simulink model "dbe_xaui_corr_32X"  (Simulink 7.1)
settings: Solver=ode45  StartTime=0.0  StopTime=1000  RelTol=1e-3
undefined symbols (not defined in the file or in its folder): iBOB
libraries: xbsIndex_r4 x455, xps_library x46, casper_library_misc x12, casper_library_sources x2, gavrt_library x1, simulink x1, casper_library_scopes x1
(part 2 of 4)

== system dbe_xaui_corr_32X/onepps_sync ==
  ext_1pps : Inport  OutDataType=sfix(16)  OutScaling=2^0
  Step : Step  Time=200  Before=1  After=0  SampleTime=1
  Terminator : Terminator
  arm1pps : xps_library/software register  Tag=xps:sw_reg  SystemSampleTime=-1  io_dir=From Processor  arith_type=Unsigned  bitwidth=32  bin_pt=0  sample_period=1  gw_name=dbe_xaui_corr_32X_onepps_sync_arm1pps_user_data_out
      link override dbe_xaui_corr_32X_onepps_sync_arm1pps_user_data_out: arith_type=Unsigned  n_bits=32  bin_pt=0  period=1
      link override dbe_xaui_corr_onepps_sync_arm1pps_user_data_out: arith_type=Unsigned  n_bits=32  bin_pt=0  period=1
      link override dbe_xaui_onepps_sync_arm1pps_user_data_out: arith_type=Unsigned  n_bits=32  bin_pt=0  period=1
      link override vlbipfb2_m3_ibob_onepps_sync_arm1pps_user_data_out: arith_type=Unsigned  n_bits=32  bin_pt=0  period=1
      link override vlbipfb2_m3_roach_onepps_sync_arm1pps_user_data_out: arith_type=Unsigned  n_bits=32  bin_pt=0  period=1
  arm1pps_ack : xps_library/software register  Tag=xps:sw_reg  SystemSampleTime=-1  io_dir=To Processor  arith_type=Unsigned  bitwidth=32  bin_pt=0  sample_period=1  gw_name=dbe_xaui_corr_32X_onepps_sync_arm1pps_ack_user_data_in
      link override convert: arith_type=Unsigned  n_bits=32  bin_pt=0
  armshake : Subsystem
  int_1pps_gen : Subsystem
  int_1pps : Outport  OutDataType=sfix(16)  OutScaling=2^0
  wires:
  int_1pps_gen/1(1pps) -> int_1pps/1
  ext_1pps/1 -> armshake/1(ext_1pps)
  arm1pps/1 -> armshake/2(ext_arm1pps)
  Step/1 -> arm1pps/1
  armshake/1(rst_1pps) -> int_1pps_gen/1(rst)
  armshake/2(arm_ack) -> arm1pps_ack/1
  arm1pps_ack/1 -> Terminator/1

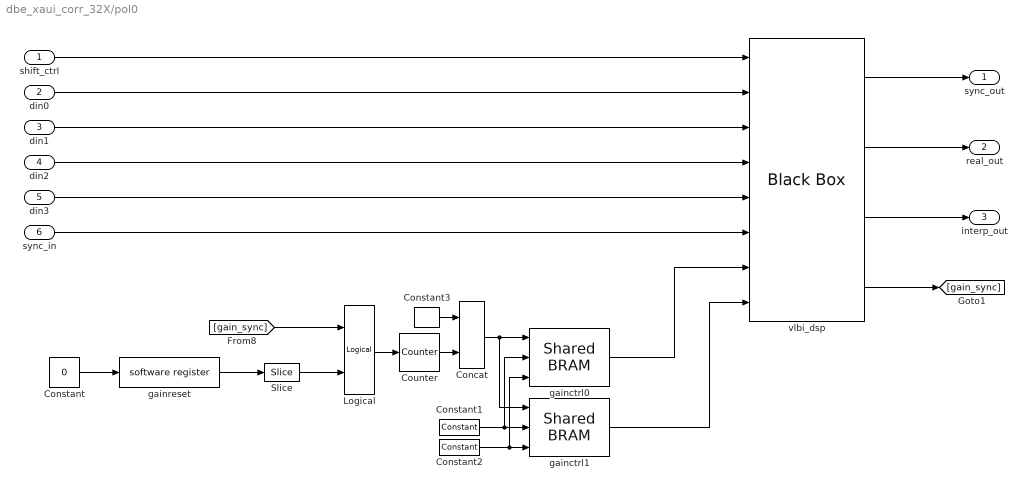
== system dbe_xaui_corr_32X/pol0 ==
  shift_ctrl : Inport  OutDataType=sfix(16)  OutScaling=2^0
  din0 : Inport  Port=2  OutDataType=sfix(16)  OutScaling=2^0
  din1 : Inport  Port=3  OutDataType=sfix(16)  OutScaling=2^0
  din2 : Inport  Port=4  OutDataType=sfix(16)  OutScaling=2^0
  din3 : Inport  Port=5  OutDataType=sfix(16)  OutScaling=2^0
  sync_in : Inport  Port=6  OutDataType=sfix(16)  OutScaling=2^0
  Concat : xbsIndex_r4/Concat  num_inputs=2  dbl_ovrd=off  block_type=concat
      settings: block_version=11.3
  Constant : Constant  Value=0  OutDataType=sfix(16)  OutScaling=2^0
  Constant1 : xbsIndex_r4/Constant  arith_type=Unsigned  const=0  n_bits=32  bin_pt=0  explicit_period=on  period=1  equ=P=C  opselect=C  inp2=PCIN>>17  opr=+  inp1=P  carry=CIN  dbl_ovrd=off  block_type=constant
      settings: block_version=11.3
  Constant2 : xbsIndex_r4/Constant  arith_type=Boolean  const=0  n_bits=1  bin_pt=0  explicit_period=on  period=1  equ=P=C  opselect=C  inp2=PCIN>>17  opr=+  inp1=P  carry=CIN  dbl_ovrd=off  block_type=constant
      settings: block_version=11.3
  Constant3 : xbsIndex_r4/Constant  arith_type=Unsigned  const=0  n_bits=8  bin_pt=0  explicit_period=on  period=1  equ=P=C  opselect=C  inp2=PCIN>>17  opr=+  inp1=P  carry=CIN  dbl_ovrd=off  block_type=constant
      settings: block_version=11.3
  Counter : xbsIndex_r4/Counter  cnt_type=Free Running  cnt_to=Inf  operation=Up  start_count=0  cnt_by_val=1  arith_type=Unsigned  n_bits=3  bin_pt=0  load_pin=off  rst=on  en=off  explicit_period=off  period=1  dbl_ovrd=off  use_behavioral_HDL=off  use_rpm=on  implementation=Fabric  block_type=counter
      settings: xl_area=[0, 0, 0, 0, 0, 0, 0]  block_version=11.3
  Logical : xbsIndex_r4/Logical  logical_function=OR  inputs=2  en=off  latency=0  precision=Full  arith_type=Unsigned  n_bits=8  bin_pt=2  align_bp=on  dbl_ovrd=off  block_type=logical
      settings: xl_area=[0, 0, 0, 0, 0, 0, 0]  block_version=11.3
  Slice : xbsIndex_r4/Slice  nbits=1  boolean_output=on  mode=Lower Bit Location + Width  bit1=0  base1=MSB of Input  bit0=0  base0=LSB of Input  dbl_ovrd=off  block_type=slice
      settings: block_version=11.3
  gainctrl0 : xps_library/Shared BRAM  Tag=xps:bram  SystemSampleTime=-1  arith_type="Signed  (2's comp)"  addr_width=11  data_width=32  data_bin_pt=0  init_vals=[0 0 100 0 zeros(1,2^11-4)]  sample_rate=1
      link override convert_din: arith_type="Signed  (2's comp)"
      link override dbe_adc_single_pol0_gainctrl0_data_out: arith_type="Signed  (2's comp)"
      link override dbe_xaui_corr_32X_pol0_gainctrl0_data_out: arith_type="Signed  (2's comp)"
      link override mem/sim_data_in: arith_type="Signed  (2's comp)"
      link override vlbipfb2_m3_ibob_pol0_gainctrl0_data_out: arith_type="Signed  (2's comp)"
      link override vlbipfb2_m3_roach_pol0_gainctrl0_data_out: arith_type="Signed  (2's comp)"
  gainctrl1 : xps_library/Shared BRAM  Tag=xps:bram  SystemSampleTime=-1  arith_type="Signed  (2's comp)"  addr_width=11  data_width=32  data_bin_pt=0  init_vals=zeros(1,2^11)  sample_rate=1
      link override convert_din: arith_type="Signed  (2's comp)"
      link override dbe_adc_single_pol0_gainctrl1_data_out: arith_type="Signed  (2's comp)"
      link override dbe_xaui_corr_32X_pol0_gainctrl1_data_out: arith_type="Signed  (2's comp)"
      link override mem/sim_data_in: arith_type="Signed  (2's comp)"
      link override vlbipfb2_m3_ibob_pol0_gainctrl1_data_out: arith_type="Signed  (2's comp)"
      link override vlbipfb2_m3_roach_pol0_gainctrl1_data_out: arith_type="Signed  (2's comp)"
  gainreset : xps_library/software register  Tag=xps:sw_reg  SystemSampleTime=-1  io_dir=From Processor  arith_type=Unsigned  bitwidth=32  bin_pt=0  sample_period=1  gw_name=dbe_xaui_corr_32X_pol0_gainreset_user_data_out
      link override dbe_adc_single_pol0_gainreset_user_data_out: arith_type=Unsigned  n_bits=32  bin_pt=0  period=1
      link override dbe_xaui_corr_32X_pol0_gainreset_user_data_out: arith_type=Unsigned  n_bits=32  bin_pt=0  period=1
      link override vlbipfb2_m3_ibob_pol0_gainreset_user_data_out: arith_type=Unsigned  n_bits=32  bin_pt=0  period=1
      link override vlbipfb2_m3_roach_pol0_gainreset_user_data_out: arith_type=Unsigned  n_bits=32  bin_pt=0  period=1
  vlbi_dsp : xbsIndex_r4/Black Box  init_code=vlbi_dsp_core_config  sim_method=Inactive  block_type=blackbox2
      settings: infoedit="Incorporates black box HDL and simulation model into a System Generator design.<P><P>You must supply a Black Box with certain information about the HDL component you would like to bring into System Generator. This information is provided through a Matlab function.<P><P>When \"Simulation mode\" is set to \"Inactive\", you will typically want to provide a separate simulation model by using a Simulation Multiplexer.<P>When \"Simulation mode\" is set to \"External co-simulator\", you must include a ModelSim block in the design."  block_version=10.1.3
  sync_out : Outport  OutDataType=sfix(16)  OutScaling=2^0
  real_out : Outport  Port=2  OutDataType=sfix(16)  OutScaling=2^0
  interp_out : Outport  Port=3  OutDataType=sfix(16)  OutScaling=2^0
  wires:
  Constant3/1 -> Concat/1
  Counter/1 -> Concat/2
  Concat/1 -> gainctrl0/1, gainctrl1/1
  Constant1/1 -> gainctrl0/2, gainctrl1/2
  Constant2/1 -> gainctrl1/3, gainctrl0/3
  Constant/1 -> gainreset/1
  Logical/1 -> Counter/1
  gainreset/1 -> Slice/1
  Slice/1 -> Logical/2
  shift_ctrl/1 -> vlbi_dsp/1
  din0/1 -> vlbi_dsp/2
  din1/1 -> vlbi_dsp/3
  din2/1 -> vlbi_dsp/4
  din3/1 -> vlbi_dsp/5
  sync_in/1 -> vlbi_dsp/6
  gainctrl0/1 -> vlbi_dsp/7
  gainctrl1/1 -> vlbi_dsp/8
  vlbi_dsp/1 -> sync_out/1
  vlbi_dsp/2 -> real_out/1
  vlbi_dsp/3 -> interp_out/1
  [gain_sync] -> Logical/1
  vlbi_dsp/4 -> [gain_sync]

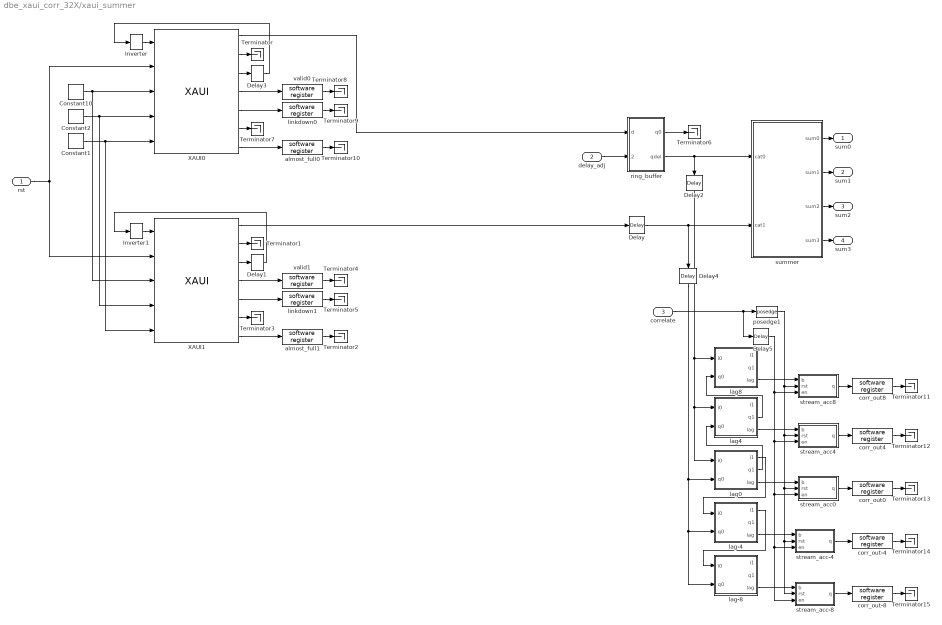
== system dbe_xaui_corr_32X/xaui_summer ==
  rst : Inport  OutDataType=sfix(16)  OutScaling=2^0
  delay_adj : Inport  Port=2  OutDataType=sfix(16)  OutScaling=2^0
  correlate : Inport  Port=3  OutDataType=sfix(16)  OutScaling=2^0
  Constant1 : xbsIndex_r4/Constant  arith_type=Boolean  const=0  n_bits=4  bin_pt=0  explicit_period=on  period=1  equ=P=C  opselect=C  inp2=PCIN>>17  opr=+  inp1=P  carry=CIN  dbl_ovrd=off  block_type=constant
      settings: block_version=11.3
  Constant10 : xbsIndex_r4/Constant  arith_type=Unsigned  const=2^4 -1  n_bits=32  bin_pt=0  explicit_period=on  period=1  equ=P=C  opselect=C  inp2=PCIN>>17  opr=+  inp1=P  carry=CIN  dbl_ovrd=off  block_type=constant
      settings: block_version=11.3
  Constant2 : xbsIndex_r4/Constant  arith_type=Unsigned  const=0  n_bits=4  bin_pt=0  explicit_period=on  period=1  equ=P=C  opselect=C  inp2=PCIN>>17  opr=+  inp1=P  carry=CIN  dbl_ovrd=off  block_type=constant
      settings: block_version=11.3
  Delay : xbsIndex_r4/Delay  en=off  latency=8  dbl_ovrd=off  reg_retiming=on  block_type=delay
  Delay1 : xbsIndex_r4/Delay  en=off  latency=32  dbl_ovrd=off  reg_retiming=off  block_type=delay
      settings: block_version=11.3
  Delay2 : xbsIndex_r4/Delay  Orientation=down  en=off  latency=8  dbl_ovrd=off  reg_retiming=on  block_type=delay
  Delay3 : xbsIndex_r4/Delay  en=off  latency=32  dbl_ovrd=off  reg_retiming=off  block_type=delay
      settings: block_version=11.3
  Delay4 : xbsIndex_r4/Delay  Orientation=down  en=off  latency=8  dbl_ovrd=off  reg_retiming=on  block_type=delay
  Delay5 : xbsIndex_r4/Delay  en=off  latency=2  dbl_ovrd=off  reg_retiming=on  block_type=delay
  Inverter : xbsIndex_r4/Inverter  en=off  latency=0  dbl_ovrd=off  block_type=inv
      settings: block_version=11.3
  Inverter1 : xbsIndex_r4/Inverter  en=off  latency=0  dbl_ovrd=off  block_type=inv
      settings: block_version=11.3
  Terminator{,1..15} (16 alike) : Terminator
  XAUI0 : xps_library/XAUI  Tag=xps:xaui  SystemSampleTime=-1  demux=2  port=iBOB:0  open_phy=off  show_param=off  pre_emph=3  swing=800
      link override convert_tx_data: n_bits=32
      link override convert_tx_outofband: n_bits=4
      link override dbe_xaui_corr_32X_xaui_summer_XAUI0_rx_data: n_bits=32
      link override dbe_xaui_corr_32X_xaui_summer_XAUI0_rx_outofband: n_bits=4
      link override dbe_xaui_corr_xaui_summer_XAUI0_rx_data: n_bits=32
      link override dbe_xaui_corr_xaui_summer_XAUI0_rx_outofband: n_bits=4
      link override dbe_xaui_xaui_summer_XAUI0_rx_data: n_bits=32
      link override dbe_xaui_xaui_summer_XAUI0_rx_outofband: n_bits=4
      link override xaui_XAUI_RECV_rx_data: n_bits=32
      link override xaui_XAUI_RECV_rx_outofband: n_bits=4
  XAUI1 : xps_library/XAUI  Tag=xps:xaui  SystemSampleTime=-1  demux=2  port=iBOB:1  open_phy=off  show_param=off  pre_emph=3  swing=800
      link override convert_tx_data: n_bits=32
      link override convert_tx_outofband: n_bits=4
      link override dbe_xaui_corr_32X_xaui_summer_XAUI1_rx_data: n_bits=32
      link override dbe_xaui_corr_32X_xaui_summer_XAUI1_rx_outofband: n_bits=4
      link override dbe_xaui_corr_xaui_summer_XAUI1_rx_data: n_bits=32
      link override dbe_xaui_corr_xaui_summer_XAUI1_rx_outofband: n_bits=4
      link override dbe_xaui_xaui_summer_XAUI1_rx_data: n_bits=32
      link override dbe_xaui_xaui_summer_XAUI1_rx_outofband: n_bits=4
      link override xaui_XAUI_RECV_rx_data: n_bits=32
      link override xaui_XAUI_RECV_rx_outofband: n_bits=4
  almost_full0 : xps_library/software register  Tag=xps:sw_reg  SystemSampleTime=-1  io_dir=To Processor  arith_type=Unsigned  bitwidth=32  bin_pt=0  sample_period=1  gw_name=dbe_xaui_corr_32X_xaui_summer_almost_full0_user_data_in
      link override convert: arith_type=Unsigned  n_bits=32  bin_pt=0
  almost_full1 : xps_library/software register  Tag=xps:sw_reg  SystemSampleTime=-1  io_dir=To Processor  arith_type=Unsigned  bitwidth=32  bin_pt=0  sample_period=1  gw_name=dbe_xaui_corr_32X_xaui_summer_almost_full1_user_data_in
      link override convert: arith_type=Unsigned  n_bits=32  bin_pt=0
  corr_out-4 : xps_library/software register  Tag=xps:sw_reg  SystemSampleTime=-1  io_dir=To Processor  arith_type="Signed  (2's comp)"  bitwidth=32  bin_pt=14  sample_period=1  gw_name=dbe_xaui_corr_32X_xaui_summer_corr_out_4_user_data_in
      link override convert: arith_type="Signed  (2's comp)"  n_bits=32  bin_pt=14
  corr_out-8 : xps_library/software register  Tag=xps:sw_reg  SystemSampleTime=-1  io_dir=To Processor  arith_type="Signed  (2's comp)"  bitwidth=32  bin_pt=14  sample_period=1  gw_name=dbe_xaui_corr_32X_xaui_summer_corr_out_8_user_data_in
      link override convert: arith_type="Signed  (2's comp)"  n_bits=32  bin_pt=14
  corr_out0 : xps_library/software register  Tag=xps:sw_reg  SystemSampleTime=-1  io_dir=To Processor  arith_type="Signed  (2's comp)"  bitwidth=32  bin_pt=14  sample_period=1  gw_name=dbe_xaui_corr_32X_xaui_summer_corr_out0_user_data_in
      link override convert: arith_type="Signed  (2's comp)"  n_bits=32  bin_pt=14
  corr_out4 : xps_library/software register  Tag=xps:sw_reg  SystemSampleTime=-1  io_dir=To Processor  arith_type="Signed  (2's comp)"  bitwidth=32  bin_pt=14  sample_period=1  gw_name=dbe_xaui_corr_32X_xaui_summer_corr_out4_user_data_in
      link override convert: arith_type="Signed  (2's comp)"  n_bits=32  bin_pt=14
  corr_out8 : xps_library/software register  Tag=xps:sw_reg  SystemSampleTime=-1  io_dir=To Processor  arith_type="Signed  (2's comp)"  bitwidth=32  bin_pt=14  sample_period=1  gw_name=dbe_xaui_corr_32X_xaui_summer_corr_out8_user_data_in
      link override convert: arith_type="Signed  (2's comp)"  n_bits=32  bin_pt=14
  lag-4 : Subsystem
  lag-8 : Subsystem
  lag0 : Subsystem
  lag4 : Subsystem
  lag8 : Subsystem
  linkdown0 : xps_library/software register  Tag=xps:sw_reg  SystemSampleTime=-1  io_dir=To Processor  arith_type=Unsigned  bitwidth=32  bin_pt=0  sample_period=1  gw_name=dbe_xaui_corr_32X_xaui_summer_linkdown0_user_data_in
      link override convert: arith_type=Unsigned  n_bits=32  bin_pt=0
  linkdown1 : xps_library/software register  Tag=xps:sw_reg  SystemSampleTime=-1  io_dir=To Processor  arith_type=Unsigned  bitwidth=32  bin_pt=0  sample_period=1  gw_name=dbe_xaui_corr_32X_xaui_summer_linkdown1_user_data_in
      link override convert: arith_type=Unsigned  n_bits=32  bin_pt=0
  posedge1 : casper_library_misc/posedge  Tag=Rising Edge Detector  SystemSampleTime=-1
  ring_buffer : Subsystem
  stream_acc-4 : Subsystem  mask{data_type=Signed, bits=32, bin_pt=14, add_latency=4}
      mask prompts: data_type "Output Data Type"; bits "Output Bit Width:"; bin_pt "Output Binary Point:"; add_latency "Adder Latency"
      mask StyleString: popup(Signed|Unsigned),edit,edit,edit
  stream_acc-8 : Subsystem  mask{data_type=Signed, bits=32, bin_pt=14, add_latency=4}
      mask prompts: data_type "Output Data Type"; bits "Output Bit Width:"; bin_pt "Output Binary Point:"; add_latency "Adder Latency"
      mask StyleString: popup(Signed|Unsigned),edit,edit,edit
  stream_acc0 : Subsystem  mask{data_type=Signed, bits=32, bin_pt=14, add_latency=4}
      mask prompts: data_type "Output Data Type"; bits "Output Bit Width:"; bin_pt "Output Binary Point:"; add_latency "Adder Latency"
      mask StyleString: popup(Signed|Unsigned),edit,edit,edit
  stream_acc4 : Subsystem  mask{data_type=Signed, bits=32, bin_pt=14, add_latency=4}
      mask prompts: data_type "Output Data Type"; bits "Output Bit Width:"; bin_pt "Output Binary Point:"; add_latency "Adder Latency"
      mask StyleString: popup(Signed|Unsigned),edit,edit,edit
  stream_acc8 : Subsystem  mask{data_type=Signed, bits=32, bin_pt=14, add_latency=4}
      mask prompts: data_type "Output Data Type"; bits "Output Bit Width:"; bin_pt "Output Binary Point:"; add_latency "Adder Latency"
      mask StyleString: popup(Signed|Unsigned),edit,edit,edit
  summer : Subsystem
  valid0 : xps_library/software register  Tag=xps:sw_reg  SystemSampleTime=-1  io_dir=To Processor  arith_type=Unsigned  bitwidth=32  bin_pt=0  sample_period=1  gw_name=dbe_xaui_corr_32X_xaui_summer_valid0_user_data_in
      link override convert: arith_type=Unsigned  n_bits=32  bin_pt=0
  valid1 : xps_library/software register  Tag=xps:sw_reg  SystemSampleTime=-1  io_dir=To Processor  arith_type=Unsigned  bitwidth=32  bin_pt=0  sample_period=1  gw_name=dbe_xaui_corr_32X_xaui_summer_valid1_user_data_in
      link override convert: arith_type=Unsigned  n_bits=32  bin_pt=0
  sum0 : Outport
  sum1 : Outport  Port=2
  sum2 : Outport  Port=3
  sum3 : Outport  Port=4
  wires:
  XAUI0/2 -> Terminator/1
  Constant2/1 -> XAUI0/4, XAUI1/4
  XAUI0/3 -> Delay3/1
  Delay3/1 -> Inverter/1
  Inverter/1 -> XAUI0/1
  XAUI0/6 -> Terminator7/1
  Constant10/1 -> XAUI0/3, XAUI1/3
  rst/1 -> XAUI0/2, XAUI1/2
  XAUI0/4 -> valid0/1
  XAUI0/5 -> linkdown0/1
  valid0/1 -> Terminator8/1
  linkdown0/1 -> Terminator9/1
  almost_full0/1 -> Terminator10/1
  XAUI0/7 -> almost_full0/1
  XAUI1/2 -> Terminator1/1
  XAUI1/3 -> Delay1/1
  Inverter1/1 -> XAUI1/1
  XAUI1/6 -> Terminator3/1
  XAUI1/4 -> valid1/1
  XAUI1/5 -> linkdown1/1
  valid1/1 -> Terminator4/1
  linkdown1/1 -> Terminator5/1
  almost_full1/1 -> Terminator2/1
  XAUI1/7 -> almost_full1/1
  Delay1/1 -> Inverter1/1
  summer/1(sum0) -> sum0/1
  summer/2(sum1) -> sum1/1
  summer/3(sum2) -> sum2/1
  summer/4(sum3) -> sum3/1
  XAUI0/1 -> ring_buffer/1(d)
  XAUI1/1 -> Delay/1
  Delay/1 -> summer/2(cat1), Delay4/1
  ring_buffer/2(qdel) -> summer/1(cat0), Delay2/1
  ring_buffer/1(q0) -> Terminator6/1
  lag0/2(q1) -> lag4/2(q0)
  lag4/2(q1) -> lag8/2(q0)
  lag0/1(i1) -> lag-4/1(i0)
  lag-4/1(i1) -> lag-8/1(i0)
  lag8/3(lag) -> stream_acc8/1(b)
  lag4/3(lag) -> stream_acc4/1(b)
  lag0/3(lag) -> stream_acc0/1(b)
  lag-8/3(lag) -> stream_acc-8/1(b)
  correlate/1 -> Delay5/1, posedge1/1
  Delay5/1 -> stream_acc-4/3(en), stream_acc-8/3(en), stream_acc0/3(en), stream_acc4/3(en), stream_acc8/3(en)
  posedge1/1 -> stream_acc-4/2(rst), stream_acc-8/2(rst), stream_acc0/2(rst), stream_acc4/2(rst), stream_acc8/2(rst)
  Constant1/1 -> XAUI0/5, XAUI1/5
  delay_adj/1 -> ring_buffer/2(delay)
  corr_out8/1 -> Terminator11/1
  stream_acc8/1(q) -> corr_out8/1
  corr_out4/1 -> Terminator12/1
  stream_acc4/1(q) -> corr_out4/1
  corr_out0/1 -> Terminator13/1
  stream_acc0/1(q) -> corr_out0/1
  corr_out-4/1 -> Terminator14/1
  stream_acc-4/1(q) -> corr_out-4/1
  corr_out-8/1 -> Terminator15/1
  stream_acc-8/1(q) -> corr_out-8/1
  lag-4/3(lag) -> stream_acc-4/1(b)
  Delay2/1 -> lag4/1(i0), lag0/1(i0), lag8/1(i0)
  Delay4/1 -> lag-4/2(q0), lag-8/2(q0), lag0/2(q0)

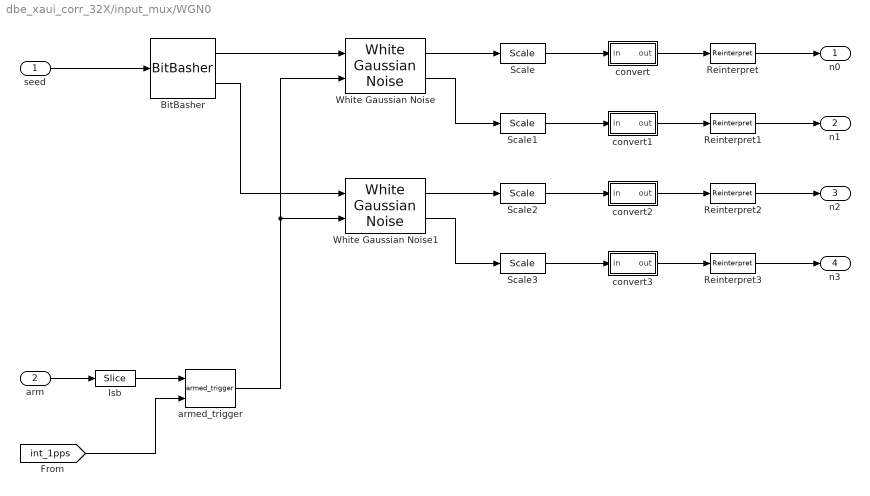
== system dbe_xaui_corr_32X/input_mux/WGN0 ==
  seed : Inport
  arm : Inport  Port=2
  BitBasher : xbsIndex_r4/BitBasher  bitexpr=|  display_expr=off  sr_1=1  arith_type1=Unsigned  bin_pt1=0  sr_2=2  arith_type2=Unsigned  bin_pt2=0  sr_3=3  arith_type3=Unsigned  bin_pt3=0  sr_4=4  arith_type4=Unsigned  bin_pt4=0  dbl_ovrd=off  block_type=bitbasher
      | <html><head><meta name="qrichtext" content="1" /><style type="text/css">
      | p, li { white-space: pre-wrap; }
      | </style></head><body style=" font-family:'MS Shell Dlg 2'; font-size:8.25pt; font-weight:400; font-style:normal;">
      | <p style=" margin-top:12px; margin-bottom:12px; margin-left:0px; margin-right:0px; -qt-block-indent:0; text-indent:0px; font-family:'MS Shell Dlg'; font-size:8pt;">s0={8'h55,s[15:0],8'haa}<br />s1={8'h55,s[31:16],8'haa}</p></body></html>
      settings: block_version=10.1.3
  Reinterpret{,1..3} (4 alike) : xbsIndex_r4/Reinterpret  force_arith_type=off  arith_type=Unsigned  force_bin_pt=on  bin_pt=7  block_type=reinterpret
      settings: infoedit="Changes signal type without altering the binary representation.   You can changed the signal between signed and unsigned, and relocate the binary point.<P><P>Hardware notes: In hardware this block costs nothing.<P><P>Example:  Suppose the input is 6 bits wide, signed, with 2 fractional bits, and the output is forced to unsigned with 0 fractional bits.  Then an input of -2.0 (1110.00 in binary 2's complement) becomes an output of 56 (111000 in binary)."  block_version=10.1.3
  Scale{,1..3} (4 alike) : xbsIndex_r4/Scale  scale_factor=4  dbl_ovrd=off  block_type=scale
      settings: infoedit=Scales input by a power of two by adjusting the binary point position.<P><P>Hardware notes: In hardware this block costs nothing.  block_version=10.1.3
  White Gaussian Noise : casper_library_sources/White Gaussian Noise  SystemSampleTime=-1  seed=hex2dec('55ffffaa')
      link override tt800_uprng/tt800_seed_gen/LFSR: rst_value='55FFFFAA'
  White Gaussian Noise1 : casper_library_sources/White Gaussian Noise  SystemSampleTime=-1  seed=hex2dec('550000aa')
      link override tt800_uprng/tt800_seed_gen/LFSR: rst_value='550000AA'
  armed_trigger : casper_library_misc/armed_trigger  SystemSampleTime=-1  hidden=0
  convert : Subsystem  AncestorBlock=casper_library/Misc/convert  mask(convert){bin_pt_in=10, n_bits_out=8, bin_pt_out=0, quantization=Round  (unbiased: +/- Inf), overflow=Wrap, latency=1}
      mask prompts: bin_pt_in "Binary Point In"; n_bits_out "Bit Width Out"; bin_pt_out "Binary Point Out"
      mask help:
      | Convert input value to the specified bit width and precision.
      |
      | Does not support upscaling number of fractional bits (eg 8_5 to 8_4 is ok, but not 8_4 to 8_5).
      mask init:
      | convert_init(gcb, ...
      |     'bin_pt_in',bin_pt_in, ...
      |     'n_bits_out',n_bits_out,...
      |     'bin_pt_out',bin_pt_out, ...
      |     'quantization',quantization,...
      |     'overflow',overflow,...
      |     'latency',latency);
      settings: AttributesFormatString=|
      | N_10 ==> 8_0
      | round inf, wrap
      | latency = 1
      mask Help:
      | <pre>
      | Description::
      | 
      | Outputs converted version of the input.
      | 
      | Mask Parameters::
      | 
      | Binary Point In (bin_pt_in): Specifies the binary point location in the input.
      | 
      | Bit Width Out (n_bits_out): Specifies the width of the output.
      | 
      | Binary Point Out (bin_pt_out): Specifies the binary point location in the output.
      | 
      | Quantization (quantization): Specifies quantization handling.
      | 
      | Overflow (overflow): Specifies overflow handling.
      | 
      | Latency (latency): Specifies the latency of the underlying adder block, which is the overall
      | latency of this block as well.
      | </pre>
      mask StyleString: edit,edit,edit,popup(Truncate|Round  (unbiased: +/- Inf)|Round  (unbiased: Even Values)|Round  (unbiased: Zero)|Round  (unbiased: Odd Values)|Round  (biased: Up)|Round  (biased: Down)),popup(Wrap|Saturate|Error),edit
  convert1 : Subsystem  AncestorBlock=casper_library/Misc/convert  mask(convert){bin_pt_in=10, n_bits_out=8, bin_pt_out=0, quantization=Round  (unbiased: +/- Inf), overflow=Wrap, latency=1}
      mask prompts: bin_pt_in "Binary Point In"; n_bits_out "Bit Width Out"; bin_pt_out "Binary Point Out"
      mask help:
      | Convert input value to the specified bit width and precision.
      |
      | Does not support upscaling number of fractional bits (eg 8_5 to 8_4 is ok, but not 8_4 to 8_5).
      mask init: same as dbe_xaui_corr_32X/input_mux/WGN0/convert
      settings: AttributesFormatString=|
      | N_10 ==> 8_0
      | round inf, wrap
      | latency = 1
      mask Help:
      | <pre>
      | Description::
      | 
      | Outputs converted version of the input.
      | 
      | Mask Parameters::
      | 
      | Binary Point In (bin_pt_in): Specifies the binary point location in the input.
      | 
      | Bit Width Out (n_bits_out): Specifies the width of the output.
      | 
      | Binary Point Out (bin_pt_out): Specifies the binary point location in the output.
      | 
      | Quantization (quantization): Specifies quantization handling.
      | 
      | Overflow (overflow): Specifies overflow handling.
      | 
      | Latency (latency): Specifies the latency of the underlying adder block, which is the overall
      | latency of this block as well.
      | </pre>
      mask StyleString: edit,edit,edit,popup(Truncate|Round  (unbiased: +/- Inf)|Round  (unbiased: Even Values)|Round  (unbiased: Zero)|Round  (unbiased: Odd Values)|Round  (biased: Up)|Round  (biased: Down)),popup(Wrap|Saturate|Error),edit
  convert2 : Subsystem  AncestorBlock=casper_library/Misc/convert  mask(convert){bin_pt_in=10, n_bits_out=8, bin_pt_out=0, quantization=Round  (unbiased: +/- Inf), overflow=Wrap, latency=1}
      mask prompts: bin_pt_in "Binary Point In"; n_bits_out "Bit Width Out"; bin_pt_out "Binary Point Out"
      mask help:
      | Convert input value to the specified bit width and precision.
      |
      | Does not support upscaling number of fractional bits (eg 8_5 to 8_4 is ok, but not 8_4 to 8_5).
      mask init: same as dbe_xaui_corr_32X/input_mux/WGN0/convert
      settings: AttributesFormatString=|
      | N_10 ==> 8_0
      | round inf, wrap
      | latency = 1
      mask Help:
      | <pre>
      | Description::
      | 
      | Outputs converted version of the input.
      | 
      | Mask Parameters::
      | 
      | Binary Point In (bin_pt_in): Specifies the binary point location in the input.
      | 
      | Bit Width Out (n_bits_out): Specifies the width of the output.
      | 
      | Binary Point Out (bin_pt_out): Specifies the binary point location in the output.
      | 
      | Quantization (quantization): Specifies quantization handling.
      | 
      | Overflow (overflow): Specifies overflow handling.
      | 
      | Latency (latency): Specifies the latency of the underlying adder block, which is the overall
      | latency of this block as well.
      | </pre>
      mask StyleString: edit,edit,edit,popup(Truncate|Round  (unbiased: +/- Inf)|Round  (unbiased: Even Values)|Round  (unbiased: Zero)|Round  (unbiased: Odd Values)|Round  (biased: Up)|Round  (biased: Down)),popup(Wrap|Saturate|Error),edit
  convert3 : Subsystem  AncestorBlock=casper_library/Misc/convert  mask(convert){bin_pt_in=10, n_bits_out=8, bin_pt_out=0, quantization=Round  (unbiased: +/- Inf), overflow=Wrap, latency=1}
      mask prompts: bin_pt_in "Binary Point In"; n_bits_out "Bit Width Out"; bin_pt_out "Binary Point Out"
      mask help:
      | Convert input value to the specified bit width and precision.
      |
      | Does not support upscaling number of fractional bits (eg 8_5 to 8_4 is ok, but not 8_4 to 8_5).
      mask init: same as dbe_xaui_corr_32X/input_mux/WGN0/convert
      settings: AttributesFormatString=|
      | N_10 ==> 8_0
      | round inf, wrap
      | latency = 1
      mask Help:
      | <pre>
      | Description::
      | 
      | Outputs converted version of the input.
      | 
      | Mask Parameters::
      | 
      | Binary Point In (bin_pt_in): Specifies the binary point location in the input.
      | 
      | Bit Width Out (n_bits_out): Specifies the width of the output.
      | 
      | Binary Point Out (bin_pt_out): Specifies the binary point location in the output.
      | 
      | Quantization (quantization): Specifies quantization handling.
      | 
      | Overflow (overflow): Specifies overflow handling.
      | 
      | Latency (latency): Specifies the latency of the underlying adder block, which is the overall
      | latency of this block as well.
      | </pre>
      mask StyleString: edit,edit,edit,popup(Truncate|Round  (unbiased: +/- Inf)|Round  (unbiased: Even Values)|Round  (unbiased: Zero)|Round  (unbiased: Odd Values)|Round  (biased: Up)|Round  (biased: Down)),popup(Wrap|Saturate|Error),edit
  lsb : xbsIndex_r4/Slice  nbits=1  boolean_output=on  mode=Lower Bit Location + Width  bit1=0  base1=MSB of Input  bit0=0  base0=LSB of Input  dbl_ovrd=off  block_type=slice
      settings: infoedit="Extracts a given range of bits from each input sample and presents it at the output.  The output type is ordinarily unsigned with binary point at zero, but can be Boolean when the slice is one bit wide.<P><P>Hardware notes: In hardware this block costs nothing."  block_version=10.1.3
  n0 : Outport
  n1 : Outport  Port=2
  n2 : Outport  Port=3
  n3 : Outport  Port=4
  wires:
  convert/1(out) -> Reinterpret/1
  Scale/1 -> convert/1(in)
  convert1/1(out) -> Reinterpret1/1
  Scale1/1 -> convert1/1(in)
  White Gaussian Noise/1 -> Scale/1
  White Gaussian Noise/2 -> Scale1/1
  Reinterpret/1 -> n0/1
  Reinterpret1/1 -> n1/1
  armed_trigger/1 -> White Gaussian Noise/2, White Gaussian Noise1/2
  arm/1 -> lsb/1
  [int_1pps] -> armed_trigger/2
  convert2/1(out) -> Reinterpret2/1
  Scale2/1 -> convert2/1(in)
  convert3/1(out) -> Reinterpret3/1
  Scale3/1 -> convert3/1(in)
  White Gaussian Noise1/1 -> Scale2/1
  White Gaussian Noise1/2 -> Scale3/1
  Reinterpret2/1 -> n2/1
  Reinterpret3/1 -> n3/1
  BitBasher/1 -> White Gaussian Noise/1
  seed/1 -> BitBasher/1
  BitBasher/2 -> White Gaussian Noise1/1
  lsb/1 -> armed_trigger/1

== system dbe_xaui_corr_32X/onepps_sync/armshake ==
  ext_1pps : Inport  OutDataType=sfix(16)  OutScaling=2^0
  ext_arm1pps : Inport  Port=2  OutDataType=sfix(16)  OutScaling=2^0
  Constant : xbsIndex_r4/Constant  arith_type=Unsigned  const=1  n_bits=1  bin_pt=0  explicit_period=on  period=1  equ=P=C  opselect=C  inp2=PCIN>>17  opr=+  inp1=P  carry=CIN  dbl_ovrd=off  block_type=constant
      settings: block_version=11.3
  Constant1 : xbsIndex_r4/Constant  arith_type=Unsigned  const=1  n_bits=1  bin_pt=0  explicit_period=on  period=1  equ=P=C  opselect=C  inp2=PCIN>>17  opr=+  inp1=P  carry=CIN  dbl_ovrd=off  block_type=constant
      settings: block_version=11.3
  Convert : xbsIndex_r4/Convert  arith_type=Boolean  n_bits=8  bin_pt=6  quantization=Truncate  overflow=Wrap  latency=0  dbl_ovrd=off  pipeline=off  block_type=convert
      settings: xl_area=[0, 0, 0, 0, 0, 0, 0]  block_version=11.3
  Convert1 : xbsIndex_r4/Convert  arith_type=Boolean  n_bits=8  bin_pt=6  quantization=Truncate  overflow=Wrap  latency=0  dbl_ovrd=off  pipeline=off  block_type=convert
      settings: xl_area=[0, 0, 0, 0, 0, 0, 0]  block_version=11.3
  Convert2 : xbsIndex_r4/Convert  arith_type=Boolean  n_bits=8  bin_pt=6  quantization=Truncate  overflow=Wrap  latency=0  dbl_ovrd=off  pipeline=off  block_type=convert
      settings: xl_area=[0, 0, 0, 0, 0, 0, 0]  block_version=11.3
  Expression : xbsIndex_r4/Expression  expression=a & ~b  align_bp=on  en=off  latency=0  precision=Full  arith_type=Unsigned  n_bits=8  bin_pt=2  dbl_ovrd=off  block_type=expr
      settings: xl_area=[0, 0, 0, 0, 0, 0, 0]  block_version=11.3
  Expression1 : xbsIndex_r4/Expression  expression=~a & b  align_bp=on  en=off  latency=0  precision=Full  arith_type=Unsigned  n_bits=8  bin_pt=2  dbl_ovrd=off  block_type=expr
      settings: xl_area=[0, 0, 0, 0, 0, 0, 0]  block_version=11.3
  Expression2 : xbsIndex_r4/Expression  expression=(a & ~b) & c  align_bp=on  en=off  latency=1  precision=Full  arith_type=Unsigned  n_bits=8  bin_pt=2  dbl_ovrd=off  block_type=expr
      settings: xl_area=[0, 0, 0, 0, 0, 0, 0]  block_version=11.3
  Register : xbsIndex_r4/Register  init=0  rst=off  en=off  dbl_ovrd=off  block_type=register
      settings: xl_area=[0, 0, 0, 0, 0, 0, 0]  block_version=11.3
  Register1 : xbsIndex_r4/Register  init=0  rst=on  en=on  dbl_ovrd=off  block_type=register
      settings: xl_area=[0, 0, 0, 0, 0, 0, 0]  block_version=11.3
  Register2 : xbsIndex_r4/Register  init=0  rst=on  en=on  dbl_ovrd=off  block_type=register
      settings: xl_area=[0, 0, 0, 0, 0, 0, 0]  block_version=11.3
  Register3 : xbsIndex_r4/Register  init=0  rst=off  en=off  dbl_ovrd=off  block_type=register
      settings: xl_area=[0, 0, 0, 0, 0, 0, 0]  block_version=11.3
  Slice8 : xbsIndex_r4/Slice  nbits=1  boolean_output=off  mode=Lower Bit Location + Width  bit1=0  base1=MSB of Input  bit0=0  base0=LSB of Input  dbl_ovrd=off  block_type=slice
      settings: block_version=11.3
  rst_1pps : Outport  OutDataType=sfix(16)  OutScaling=2^0
  arm_ack : Outport  Port=2  OutDataType=sfix(16)  OutScaling=2^0
  wires:
  Register/1 -> Expression/2, Expression1/2
  Convert/1 -> Expression2/3
  Register3/1 -> Expression2/2
  Slice8/1 -> Expression/1, Register/1, Expression1/1
  Register1/1 -> Convert/1
  ext_1pps/1 -> Expression2/1, Register3/1
  Expression2/1 -> rst_1pps/1, Register1/2, Register2/3
  ext_arm1pps/1 -> Slice8/1
  Constant/1 -> Register1/1
  Expression/1 -> Convert1/1
  Constant1/1 -> Register2/1
  Expression1/1 -> Convert2/1
  Register2/1 -> arm_ack/1
  Convert1/1 -> Register1/3
  Convert2/1 -> Register2/2

== system dbe_xaui_corr_32X/onepps_sync/int_1pps_gen ==
  rst : Inport  OutDataType=sfix(16)  OutScaling=2^0
  1pps_gen : Subsystem
  Simulation Multiplexer : xbsIndex_r4/Simulation Multiplexer  sim_sel=2  hw_sel=1  block_type=simmux
      settings: infoedit="Distinguish input subsystems as \"simulation only\" and \"generation only\".  The input specified For Simulation will be used during Simulink simulation.  The input specified For Generation will be used during code generation.  This block will typically be used on the output of a HW Co-Simulation, Black Box, or ModelSim subsystem.<br><br>Hardware Notes: This block costs nothing."  block_version=11.3
  sim1pps_gen : Subsystem
  1pps : Outport  OutDataType=sfix(16)  OutScaling=2^0
  wires:
  Simulation Multiplexer/1 -> 1pps/1
  rst/1 -> sim1pps_gen/1(rst), 1pps_gen/1(rst)
  sim1pps_gen/1(1pps_sim) -> Simulation Multiplexer/2
  1pps_gen/1(1pps) -> Simulation Multiplexer/1

== system dbe_xaui_corr_32X/xaui_summer/lag-4 ==
  i0 : Inport  OutDataType=sfix(16)  OutScaling=2^0
  q0 : Inport  Port=2  OutDataType=sfix(16)  OutScaling=2^0
  AddSub : xbsIndex_r4/AddSub  mode=Addition  use_carryin=off  use_carryout=off  en=off  latency=2  precision=Full  arith_type=Unsigned  n_bits=16  bin_pt=14  quantization=Truncate  overflow=Wrap  dbl_ovrd=off  use_behavioral_HDL=off  pipelined=off  use_rpm=on  hw_selection=Fabric  block_type=addsub
      settings: block_version=10.1.3
  AddSub1 : xbsIndex_r4/AddSub  mode=Addition  use_carryin=off  use_carryout=off  en=off  latency=2  precision=Full  arith_type=Unsigned  n_bits=16  bin_pt=14  quantization=Truncate  overflow=Wrap  dbl_ovrd=off  use_behavioral_HDL=off  pipelined=off  use_rpm=on  hw_selection=Fabric  block_type=addsub
      settings: block_version=10.1.3
  AddSub2 : xbsIndex_r4/AddSub  mode=Addition  use_carryin=off  use_carryout=off  en=off  latency=2  precision=Full  arith_type=Unsigned  n_bits=16  bin_pt=14  quantization=Truncate  overflow=Wrap  dbl_ovrd=off  use_behavioral_HDL=off  pipelined=off  use_rpm=on  hw_selection=Fabric  block_type=addsub
      settings: block_version=10.1.3
  Delay : xbsIndex_r4/Delay  en=off  latency=1  dbl_ovrd=off  reg_retiming=off  block_type=delay
  Delay1 : xbsIndex_r4/Delay  en=off  latency=1  dbl_ovrd=off  reg_retiming=off  block_type=delay
  Mult{,1..3} (4 alike) : xbsIndex_r4/Mult  precision=Full  arith_type="Signed  (2's comp)"  n_bits=16  bin_pt=14  quantization=Truncate  overflow=Wrap  en=off  latency=5  dbl_ovrd=off  use_behavioral_HDL=on  use_embedded=off  opt=Speed  optimum_pipeline=on  pipeline=on  use_rpm=on  placement_style=Triangular  block_type=mult
      settings: infoedit=Hardware notes: To use the internal pipeline stage of the dedicated multiplier you must select 'Pipeline for maximum performance'.  block_version=10.1.3
  uncram : Subsystem  AncestorBlock=gavrt_library/uncram  mask(uncram){num_slice=4, slice_width=8, bin_pt=7, arith_type=1}
      mask prompts: num_slice "Number of slices"; slice_width "Slice Width"; bin_pt "Output Binary Point"; arith_type "Output Arithmetic Type (0=Unsigned, 1=Signed)"
      mask help: Takes a concatenated input and slices it up into even pieces and reinterprets them as signed fixed point numbers with a given binary point.
      mask init:
      | uncram_init(gcb, ...
      |     'num_slice', num_slice, ...
      |     'slice_width', slice_width, ...
      |     'bin_pt', bin_pt, ...
      |     'arith_type', arith_type);
      settings: AttributesFormatString=Fix_8_7
  uncram1 : Subsystem  AncestorBlock=gavrt_library/uncram  mask(uncram){num_slice=4, slice_width=8, bin_pt=7, arith_type=1}
      mask prompts: num_slice "Number of slices"; slice_width "Slice Width"; bin_pt "Output Binary Point"; arith_type "Output Arithmetic Type (0=Unsigned, 1=Signed)"
      mask help: Takes a concatenated input and slices it up into even pieces and reinterprets them as signed fixed point numbers with a given binary point.
      mask init:
      | uncram_init(gcb, ...
      |     'num_slice', num_slice, ...
      |     'slice_width', slice_width, ...
      |     'bin_pt', bin_pt, ...
      |     'arith_type', arith_type);
      settings: AttributesFormatString=Fix_8_7
  i1 : Outport  OutDataType=sfix(16)  OutScaling=2^0
  q1 : Outport  Port=2  OutDataType=sfix(16)  OutScaling=2^0
  lag : Outport  Port=3  OutDataType=sfix(16)  OutScaling=2^0
  wires:
  AddSub2/1 -> lag/1
  AddSub1/1 -> AddSub2/2
  AddSub/1 -> AddSub2/1
  Mult3/1 -> AddSub1/2
  Mult2/1 -> AddSub1/1
  Mult1/1 -> AddSub/2
  Mult/1 -> AddSub/1
  uncram1/4(Out4) -> Mult3/2
  uncram1/3(Out3) -> Mult2/2
  uncram1/2(Out2) -> Mult1/2
  uncram1/1(Out1) -> Mult/2
  uncram/4(Out4) -> Mult3/1
  uncram/3(Out3) -> Mult2/1
  uncram/2(Out2) -> Mult1/1
  uncram/1(Out1) -> Mult/1
  Delay1/1 -> q1/1
  Delay/1 -> i1/1
  q0/1 -> Delay1/1, uncram1/1(In)
  i0/1 -> Delay/1, uncram/1(In)

== system dbe_xaui_corr_32X/xaui_summer/lag-8 ==
  i0 : Inport  OutDataType=sfix(16)  OutScaling=2^0
  q0 : Inport  Port=2  OutDataType=sfix(16)  OutScaling=2^0
  AddSub : xbsIndex_r4/AddSub  mode=Addition  use_carryin=off  use_carryout=off  en=off  latency=2  precision=Full  arith_type=Unsigned  n_bits=16  bin_pt=14  quantization=Truncate  overflow=Wrap  dbl_ovrd=off  use_behavioral_HDL=off  pipelined=off  use_rpm=on  hw_selection=Fabric  block_type=addsub
      settings: block_version=10.1.3
  AddSub1 : xbsIndex_r4/AddSub  mode=Addition  use_carryin=off  use_carryout=off  en=off  latency=2  precision=Full  arith_type=Unsigned  n_bits=16  bin_pt=14  quantization=Truncate  overflow=Wrap  dbl_ovrd=off  use_behavioral_HDL=off  pipelined=off  use_rpm=on  hw_selection=Fabric  block_type=addsub
      settings: block_version=10.1.3
  AddSub2 : xbsIndex_r4/AddSub  mode=Addition  use_carryin=off  use_carryout=off  en=off  latency=2  precision=Full  arith_type=Unsigned  n_bits=16  bin_pt=14  quantization=Truncate  overflow=Wrap  dbl_ovrd=off  use_behavioral_HDL=off  pipelined=off  use_rpm=on  hw_selection=Fabric  block_type=addsub
      settings: block_version=10.1.3
  Delay : xbsIndex_r4/Delay  en=off  latency=1  dbl_ovrd=off  reg_retiming=off  block_type=delay
  Delay1 : xbsIndex_r4/Delay  en=off  latency=1  dbl_ovrd=off  reg_retiming=off  block_type=delay
  Mult{,1..3} (4 alike) : xbsIndex_r4/Mult  precision=Full  arith_type="Signed  (2's comp)"  n_bits=16  bin_pt=14  quantization=Truncate  overflow=Wrap  en=off  latency=5  dbl_ovrd=off  use_behavioral_HDL=on  use_embedded=off  opt=Speed  optimum_pipeline=on  pipeline=on  use_rpm=on  placement_style=Triangular  block_type=mult
      settings: infoedit=Hardware notes: To use the internal pipeline stage of the dedicated multiplier you must select 'Pipeline for maximum performance'.  block_version=10.1.3
  uncram : Subsystem  AncestorBlock=gavrt_library/uncram  mask(uncram){num_slice=4, slice_width=8, bin_pt=7, arith_type=1}
      mask prompts: num_slice "Number of slices"; slice_width "Slice Width"; bin_pt "Output Binary Point"; arith_type "Output Arithmetic Type (0=Unsigned, 1=Signed)"
      mask help: Takes a concatenated input and slices it up into even pieces and reinterprets them as signed fixed point numbers with a given binary point.
      mask init:
      | uncram_init(gcb, ...
      |     'num_slice', num_slice, ...
      |     'slice_width', slice_width, ...
      |     'bin_pt', bin_pt, ...
      |     'arith_type', arith_type);
      settings: AttributesFormatString=Fix_8_7
  uncram1 : Subsystem  AncestorBlock=gavrt_library/uncram  mask(uncram){num_slice=4, slice_width=8, bin_pt=7, arith_type=1}
      mask prompts: num_slice "Number of slices"; slice_width "Slice Width"; bin_pt "Output Binary Point"; arith_type "Output Arithmetic Type (0=Unsigned, 1=Signed)"
      mask help: Takes a concatenated input and slices it up into even pieces and reinterprets them as signed fixed point numbers with a given binary point.
      mask init:
      | uncram_init(gcb, ...
      |     'num_slice', num_slice, ...
      |     'slice_width', slice_width, ...
      |     'bin_pt', bin_pt, ...
      |     'arith_type', arith_type);
      settings: AttributesFormatString=Fix_8_7
  i1 : Outport  OutDataType=sfix(16)  OutScaling=2^0
  q1 : Outport  Port=2  OutDataType=sfix(16)  OutScaling=2^0
  lag : Outport  Port=3  OutDataType=sfix(16)  OutScaling=2^0
  wires:
  i0/1 -> uncram/1(In), Delay/1
  q0/1 -> uncram1/1(In), Delay1/1
  Delay/1 -> i1/1
  Delay1/1 -> q1/1
  uncram/1(Out1) -> Mult/1
  uncram/2(Out2) -> Mult1/1
  uncram/3(Out3) -> Mult2/1
  uncram/4(Out4) -> Mult3/1
  uncram1/1(Out1) -> Mult/2
  uncram1/2(Out2) -> Mult1/2
  uncram1/3(Out3) -> Mult2/2
  uncram1/4(Out4) -> Mult3/2
  Mult/1 -> AddSub/1
  Mult1/1 -> AddSub/2
  Mult2/1 -> AddSub1/1
  Mult3/1 -> AddSub1/2
  AddSub/1 -> AddSub2/1
  AddSub1/1 -> AddSub2/2
  AddSub2/1 -> lag/1

== system dbe_xaui_corr_32X/xaui_summer/lag0 ==
  i0 : Inport  OutDataType=sfix(16)  OutScaling=2^0
  q0 : Inport  Port=2  OutDataType=sfix(16)  OutScaling=2^0
  AddSub : xbsIndex_r4/AddSub  mode=Addition  use_carryin=off  use_carryout=off  en=off  latency=2  precision=Full  arith_type=Unsigned  n_bits=16  bin_pt=14  quantization=Truncate  overflow=Wrap  dbl_ovrd=off  use_behavioral_HDL=off  pipelined=off  use_rpm=on  hw_selection=Fabric  block_type=addsub
      settings: block_version=10.1.3
  AddSub1 : xbsIndex_r4/AddSub  mode=Addition  use_carryin=off  use_carryout=off  en=off  latency=2  precision=Full  arith_type=Unsigned  n_bits=16  bin_pt=14  quantization=Truncate  overflow=Wrap  dbl_ovrd=off  use_behavioral_HDL=off  pipelined=off  use_rpm=on  hw_selection=Fabric  block_type=addsub
      settings: block_version=10.1.3
  AddSub2 : xbsIndex_r4/AddSub  mode=Addition  use_carryin=off  use_carryout=off  en=off  latency=2  precision=Full  arith_type=Unsigned  n_bits=16  bin_pt=14  quantization=Truncate  overflow=Wrap  dbl_ovrd=off  use_behavioral_HDL=off  pipelined=off  use_rpm=on  hw_selection=Fabric  block_type=addsub
      settings: block_version=10.1.3
  Delay : xbsIndex_r4/Delay  en=off  latency=1  dbl_ovrd=off  reg_retiming=off  block_type=delay
  Delay1 : xbsIndex_r4/Delay  en=off  latency=1  dbl_ovrd=off  reg_retiming=off  block_type=delay
  Mult{,1..3} (4 alike) : xbsIndex_r4/Mult  precision=Full  arith_type="Signed  (2's comp)"  n_bits=16  bin_pt=14  quantization=Truncate  overflow=Wrap  en=off  latency=5  dbl_ovrd=off  use_behavioral_HDL=on  use_embedded=off  opt=Speed  optimum_pipeline=on  pipeline=on  use_rpm=on  placement_style=Triangular  block_type=mult
      settings: infoedit=Hardware notes: To use the internal pipeline stage of the dedicated multiplier you must select 'Pipeline for maximum performance'.  block_version=10.1.3
  uncram : Subsystem  AncestorBlock=gavrt_library/uncram  mask(uncram){num_slice=4, slice_width=8, bin_pt=7, arith_type=1}
      mask prompts: num_slice "Number of slices"; slice_width "Slice Width"; bin_pt "Output Binary Point"; arith_type "Output Arithmetic Type (0=Unsigned, 1=Signed)"
      mask help: Takes a concatenated input and slices it up into even pieces and reinterprets them as signed fixed point numbers with a given binary point.
      mask init:
      | uncram_init(gcb, ...
      |     'num_slice', num_slice, ...
      |     'slice_width', slice_width, ...
      |     'bin_pt', bin_pt, ...
      |     'arith_type', arith_type);
      settings: AttributesFormatString=Fix_8_7
  uncram1 : Subsystem  AncestorBlock=gavrt_library/uncram  mask(uncram){num_slice=4, slice_width=8, bin_pt=7, arith_type=1}
      mask prompts: num_slice "Number of slices"; slice_width "Slice Width"; bin_pt "Output Binary Point"; arith_type "Output Arithmetic Type (0=Unsigned, 1=Signed)"
      mask help: Takes a concatenated input and slices it up into even pieces and reinterprets them as signed fixed point numbers with a given binary point.
      mask init:
      | uncram_init(gcb, ...
      |     'num_slice', num_slice, ...
      |     'slice_width', slice_width, ...
      |     'bin_pt', bin_pt, ...
      |     'arith_type', arith_type);
      settings: AttributesFormatString=Fix_8_7
  i1 : Outport  OutDataType=sfix(16)  OutScaling=2^0
  q1 : Outport  Port=2  OutDataType=sfix(16)  OutScaling=2^0
  lag : Outport  Port=3  OutDataType=sfix(16)  OutScaling=2^0
  wires:
  i0/1 -> uncram/1(In), Delay/1
  q0/1 -> uncram1/1(In), Delay1/1
  Delay/1 -> i1/1
  Delay1/1 -> q1/1
  uncram/1(Out1) -> Mult/1
  uncram/2(Out2) -> Mult1/1
  uncram/3(Out3) -> Mult2/1
  uncram/4(Out4) -> Mult3/1
  uncram1/1(Out1) -> Mult/2
  uncram1/2(Out2) -> Mult1/2
  uncram1/3(Out3) -> Mult2/2
  uncram1/4(Out4) -> Mult3/2
  Mult/1 -> AddSub/1
  Mult1/1 -> AddSub/2
  Mult2/1 -> AddSub1/1
  Mult3/1 -> AddSub1/2
  AddSub/1 -> AddSub2/1
  AddSub1/1 -> AddSub2/2
  AddSub2/1 -> lag/1

== system dbe_xaui_corr_32X/xaui_summer/lag4 ==
  i0 : Inport  OutDataType=sfix(16)  OutScaling=2^0
  q0 : Inport  Port=2  OutDataType=sfix(16)  OutScaling=2^0
  AddSub : xbsIndex_r4/AddSub  mode=Addition  use_carryin=off  use_carryout=off  en=off  latency=2  precision=Full  arith_type=Unsigned  n_bits=16  bin_pt=14  quantization=Truncate  overflow=Wrap  dbl_ovrd=off  use_behavioral_HDL=off  pipelined=off  use_rpm=on  hw_selection=Fabric  block_type=addsub
      settings: block_version=10.1.3
  AddSub1 : xbsIndex_r4/AddSub  mode=Addition  use_carryin=off  use_carryout=off  en=off  latency=2  precision=Full  arith_type=Unsigned  n_bits=16  bin_pt=14  quantization=Truncate  overflow=Wrap  dbl_ovrd=off  use_behavioral_HDL=off  pipelined=off  use_rpm=on  hw_selection=Fabric  block_type=addsub
      settings: block_version=10.1.3
  AddSub2 : xbsIndex_r4/AddSub  mode=Addition  use_carryin=off  use_carryout=off  en=off  latency=2  precision=Full  arith_type=Unsigned  n_bits=16  bin_pt=14  quantization=Truncate  overflow=Wrap  dbl_ovrd=off  use_behavioral_HDL=off  pipelined=off  use_rpm=on  hw_selection=Fabric  block_type=addsub
      settings: block_version=10.1.3
  Delay : xbsIndex_r4/Delay  en=off  latency=1  dbl_ovrd=off  reg_retiming=off  block_type=delay
  Delay1 : xbsIndex_r4/Delay  en=off  latency=1  dbl_ovrd=off  reg_retiming=off  block_type=delay
  Mult{,1..3} (4 alike) : xbsIndex_r4/Mult  precision=Full  arith_type="Signed  (2's comp)"  n_bits=16  bin_pt=14  quantization=Truncate  overflow=Wrap  en=off  latency=5  dbl_ovrd=off  use_behavioral_HDL=on  use_embedded=off  opt=Speed  optimum_pipeline=on  pipeline=on  use_rpm=on  placement_style=Triangular  block_type=mult
      settings: infoedit=Hardware notes: To use the internal pipeline stage of the dedicated multiplier you must select 'Pipeline for maximum performance'.  block_version=10.1.3
  uncram : Subsystem  AncestorBlock=gavrt_library/uncram  mask(uncram){num_slice=4, slice_width=8, bin_pt=7, arith_type=1}
      mask prompts: num_slice "Number of slices"; slice_width "Slice Width"; bin_pt "Output Binary Point"; arith_type "Output Arithmetic Type (0=Unsigned, 1=Signed)"
      mask help: Takes a concatenated input and slices it up into even pieces and reinterprets them as signed fixed point numbers with a given binary point.
      mask init:
      | uncram_init(gcb, ...
      |     'num_slice', num_slice, ...
      |     'slice_width', slice_width, ...
      |     'bin_pt', bin_pt, ...
      |     'arith_type', arith_type);
      settings: AttributesFormatString=Fix_8_7
  uncram1 : Subsystem  AncestorBlock=gavrt_library/uncram  mask(uncram){num_slice=4, slice_width=8, bin_pt=7, arith_type=1}
      mask prompts: num_slice "Number of slices"; slice_width "Slice Width"; bin_pt "Output Binary Point"; arith_type "Output Arithmetic Type (0=Unsigned, 1=Signed)"
      mask help: Takes a concatenated input and slices it up into even pieces and reinterprets them as signed fixed point numbers with a given binary point.
      mask init:
      | uncram_init(gcb, ...
      |     'num_slice', num_slice, ...
      |     'slice_width', slice_width, ...
      |     'bin_pt', bin_pt, ...
      |     'arith_type', arith_type);
      settings: AttributesFormatString=Fix_8_7
  i1 : Outport  OutDataType=sfix(16)  OutScaling=2^0
  q1 : Outport  Port=2  OutDataType=sfix(16)  OutScaling=2^0
  lag : Outport  Port=3  OutDataType=sfix(16)  OutScaling=2^0
  wires:
  AddSub2/1 -> lag/1
  AddSub1/1 -> AddSub2/2
  AddSub/1 -> AddSub2/1
  Mult3/1 -> AddSub1/2
  Mult2/1 -> AddSub1/1
  Mult1/1 -> AddSub/2
  Mult/1 -> AddSub/1
  uncram1/4(Out4) -> Mult3/2
  uncram1/3(Out3) -> Mult2/2
  uncram1/2(Out2) -> Mult1/2
  uncram1/1(Out1) -> Mult/2
  uncram/4(Out4) -> Mult3/1
  uncram/3(Out3) -> Mult2/1
  uncram/2(Out2) -> Mult1/1
  uncram/1(Out1) -> Mult/1
  Delay1/1 -> q1/1
  Delay/1 -> i1/1
  q0/1 -> Delay1/1, uncram1/1(In)
  i0/1 -> Delay/1, uncram/1(In)
